simulink model "Nx8000_c"  (R2022b)
settings: Solver=VariableStepAuto  StartTime=0.0  StopTime=inf  RelTol=1e-3
libraries: instrumentseriallib x3
settings Model: Creator=twopi  LastModifiedBy=twopi

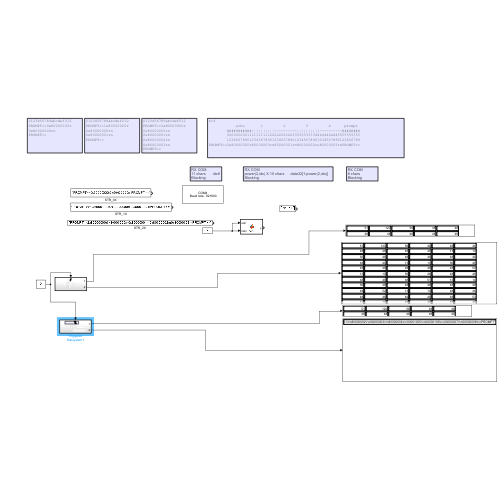
[thumbnail: Simulink's stored preview of the top-level diagram]
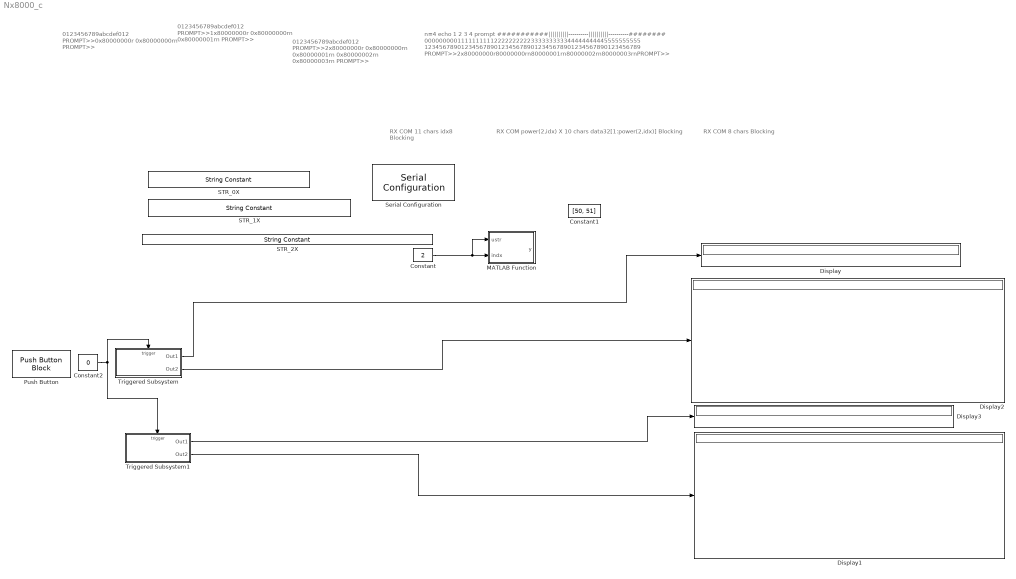
== system Nx8000_c ==
  note: RX COM
      | 11 chars       idx8
      | Blocking
  note: 0123456789abcdef012
      | PROMPT>>0x80000000r
      | 0x80000000rn
      | PROMPT>>
  note: 0123456789abcdef012
      | PROMPT>>1x80000000r
      | 0x80000000rn
      | 0x80000001rn
      | PROMPT>>
  note: 0123456789abcdef012
      | PROMPT>>2x80000000r
      | 0x80000000rn
      | 0x80000001rn
      | 0x80000002rn
      | 0x80000003rn
      | PROMPT>>
  note: n=4
      |             echo       1         2         3         4      prompt
      |         ###########||||||||||----------||||||||||----------########
      |         00000000011111111112222222222333333333344444444445555555555
      |         12345678901234567890123456789012345678901234567890123456789
      | PROMPT>>2x80000000r80000000rn80000001rn80000002rn80000003rnPROMPT>>
  note: RX COM
      | power(2,idx) X 10 chars      data32[1:power(2,idx)]
      | Blocking
  note: RX COM
      | 8 chars
      | Blocking
  Constant : Constant  Value=2  OutDataTypeStr=uint8
  Constant1 : Constant  Value=[50, 51]  OutDataTypeStr=uint8
  Constant2 : Constant  Value=0  OutDataTypeStr=uint8  SampleTime=Inf
  Display{,1..3} (4 alike) : Display
  MATLAB Function : MATLAB Function  TreatAsAtomicUnit=on
  Push Button : PushButtonBlock  OffValue=0.000000
  STR_0X : StringConstant  String="\"PROMPT>>0x80000000r0x80000000rnPROMPT>>\""
  STR_1X : StringConstant  String="\"PROMPT>>1x80000000r0x80000000rn0x80000001rnPROMPT>>\""
  STR_2X : StringConstant  String="\"PROMPT>>2x80000000r0x80000000rn0x80000001rn0x80000002rn0x80000003rnPROMPT>>\""
  Serial Configuration : instrumentseriallib/Serial Configuration  Priority=-200000  PortSel=COM4  Port=COM4  ComPort=COM4  BaudRate=921600  DataBits=8  Parity=none  StopBits=1  ByteOrder=little-endian  FlowControl=none  Timeout=10  SimulateUsing=Interpreted execution  BlockInModel=on  aMode=1
  Triggered Subsystem : Subsystem  TreatAsAtomicUnit=on
      settings: LibrarySourceBlock=|
      | hdlsllib/Ports &
      | Subsystems/Triggered
      | Subsystem
  Triggered Subsystem1 : Subsystem  TreatAsAtomicUnit=on
      settings: LibrarySourceBlock=|
      | hdlsllib/Ports &
      | Subsystems/Triggered
      | Subsystem
  wires:
  Constant/1 -> MATLAB Function/1(ustr), MATLAB Function/2(indx)
  Triggered Subsystem/1(Out1) -> Display/1
  Constant2/1 -> Triggered Subsystem1/Trigger, Triggered Subsystem/Trigger
  Triggered Subsystem1/1(Out1) -> Display3/1
  Triggered Subsystem/2(Out2) -> Display2/1
  Triggered Subsystem1/2(Out2) -> Display1/1

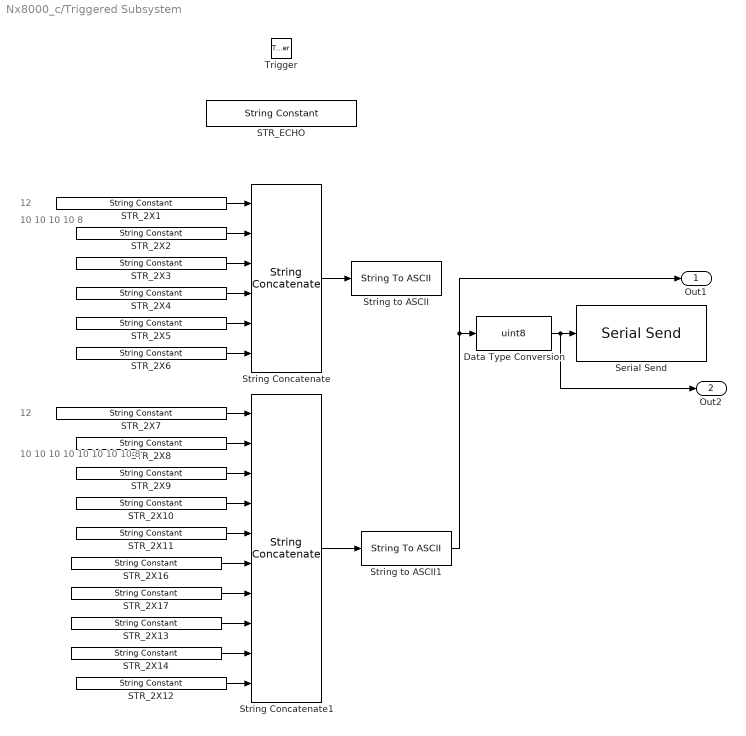
== system Nx8000_c/Triggered Subsystem ==
  note: 12
  note: 10
      |
      | 10
      |
      |
      | 10
      |
      | 10
      |
      | 8
  note: 12
  note: 10
      |
      | 10
      |
      |
      | 10
      |
      | 10
      |
      | 10
      |
      | 10
      |
      |
      | 10
      |
      | 10
      |
      | 8
  Trigger : TriggerPort  VariantControl=(inherit)
  Data Type Conversion : DataTypeConversion  OutDataTypeStr=uint8  SaturateOnIntegerOverflow=off  RndMeth=Floor
  STR_2X1 : StringConstant  String="\"2x80000000\"+char(13)+char(10)"
  STR_2X10 : StringConstant  String="\"80000003\"+char(13)+char(10)"
  STR_2X11 : StringConstant  String="\"80000004\"+char(13)+char(10)"
  STR_2X12 : StringConstant  String="\"PROMPT>>\""
  STR_2X13 : StringConstant  String="\"00000007\"+char(13)+char(10)"
  STR_2X14 : StringConstant  String="\"00000008\"+char(13)+char(10)"
  STR_2X16 : StringConstant  String="\"00001005\"+char(13)+char(10)"
  STR_2X17 : StringConstant  String="\"00000106\"+char(13)+char(10)"
  STR_2X2 : StringConstant  String="\"80000001\"+char(13)+char(10)"
  STR_2X3 : StringConstant  String="\"80000002\"+char(13)+char(10)"
  STR_2X4 : StringConstant  String="\"80000003\"+char(13)+char(10)"
  STR_2X5 : StringConstant  String="\"80000004\"+char(13)+char(10)"
  STR_2X6 : StringConstant  String="\"PROMPT>>\""
  STR_2X7 : StringConstant  String="\"3x80000000\"+char(13)+char(10)"
  STR_2X8 : StringConstant  String="\"80000001\"+char(13)+char(10)"
  STR_2X9 : StringConstant  String="\"80000002\"+char(13)+char(10)"
  STR_ECHO : StringConstant  String="\"0x8765\" + \"4321\""
  Serial Send : instrumentseriallib/Serial Send  Priority=1  PortSel=COM4  Port=COM4  ComPort=COM4  Header=[]  Terminator=Custom terminator  CustomTerminator=[62, 62]  EnableBlockingMode=on  SimulateUsing=Interpreted execution  BlockInModel=on  aMode=1
  String Concatenate : StringConcatenate  Inputs=6
  String Concatenate1 : StringConcatenate  Inputs=10
  String to ASCII : StringToASCII  OutputVectorSize=60
  String to ASCII1 : StringToASCII  OutputVectorSize=100
  Out1 : Outport
  Out2 : Outport  Port=2
  wires:
  STR_2X1/1 -> String Concatenate/1
  STR_2X2/1 -> String Concatenate/2
  STR_2X3/1 -> String Concatenate/3
  STR_2X4/1 -> String Concatenate/4
  STR_2X5/1 -> String Concatenate/5
  STR_2X6/1 -> String Concatenate/6
  Data Type Conversion/1 -> Out2/1, Serial Send/1
  STR_2X9/1 -> String Concatenate1/3
  STR_2X8/1 -> String Concatenate1/2
  STR_2X11/1 -> String Concatenate1/5
  STR_2X10/1 -> String Concatenate1/4
  STR_2X7/1 -> String Concatenate1/1
  STR_2X12/1 -> String Concatenate1/10
  STR_2X14/1 -> String Concatenate1/9
  STR_2X13/1 -> String Concatenate1/8
  STR_2X17/1 -> String Concatenate1/7
  STR_2X16/1 -> String Concatenate1/6
  String Concatenate1/1 -> String to ASCII1/1
  String to ASCII1/1 -> Out1/1, Data Type Conversion/1
  String Concatenate/1 -> String to ASCII/1

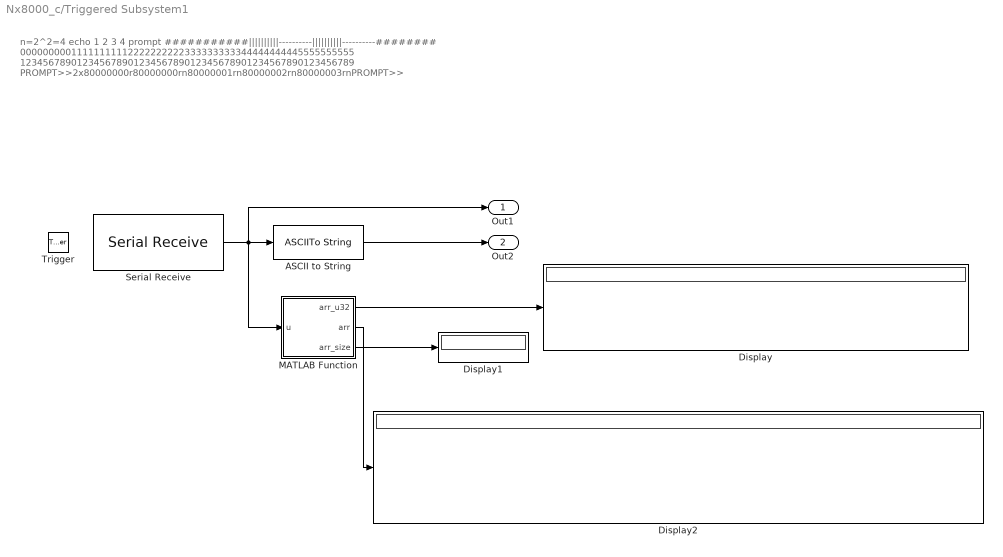
== system Nx8000_c/Triggered Subsystem1 ==
  note: n=2^2=4
      |             echo       1         2         3         4      prompt
      |         ###########||||||||||----------||||||||||----------########
      |         00000000011111111112222222222333333333344444444445555555555
      |         12345678901234567890123456789012345678901234567890123456789
      | PROMPT>>2x80000000r80000000rn80000001rn80000002rn80000003rnPROMPT>>
  Trigger : TriggerPort  TriggerType=falling  VariantControl=(inherit)
  ASCII to String : ASCIIToString
  Display : Display
  Display1 : Display
  Display2 : Display
  MATLAB Function : MATLAB Function  TreatAsAtomicUnit=on
  Serial Receive : instrumentseriallib/Serial Receive  Priority=1  PortSel=COM4  Port=COM4  ComPort=COM4  DataType=uint8  SaveDataType=uint8  ToggleHeader=off  Header=[]  ToggleTerminator=on  Terminator=Custom terminator  CustomTerminator=[62, 62]  InputFormat=Column major  ToggleDataSize=on  DataSize=[1 98]  EnableBlockingMode=on  ActionDataUnavailable=Output last received value  ActionWhenDataUnavailable=Output last received value  CustomValue=0  SampleTime=-1  SimulateUsing=Interpreted execution  BlockInModel=on  aMode=1
  Out1 : Outport
  Out2 : Outport  Port=2
  wires:
  Serial Receive/1 -> MATLAB Function/1(u), Out1/1, ASCII to String/1
  ASCII to String/1 -> Out2/1
  MATLAB Function/2(arr) -> Display2/1
  MATLAB Function/1(arr_u32) -> Display/1
  MATLAB Function/3(arr_size) -> Display1/1

== matlab function Nx8000_c/Triggered Subsystem1/MATLAB Function ==
  data: u input; arr_u32 output; arr output; arr_size output
function [arr_u32, arr, arr_size]    = fcn(u)

  nmax      = 2^8;

  arr       = zeros(nmax,8);     % create empty array of uint8 array
  arr_u32   = zeros(nmax,1);     % create empty array of uint32
  arr_size  = 2^(char(u(1))-48); % get an output arr size from ECHO (Header)

  arr_c     = char(u);           % cast input STRING into UINT8 array
  arr_u8    = uint8(arr_c);      % cast input STRING into UINT8 array

%KEEP echo  = arr_c(1,1:12);    % echo is dropped

  for i = 1 : arr_size
    arr     (i,:) = arr_u8(13+10*(i-1):20+10*(i-1)); % data only
    arr_cc        = arr_c (13+10*(i-1):20+10*(i-1)); % data only
    arr_u32 (i,1) = uint32(hex2dec(string(arr_cc))); % data only
  end

 %  arr_u32(1:arr_size,:) = arr_u32(1:nmax,:); % data only


end

== matlab function Nx8000_c/MATLAB Function ==
  data: ustr input; y output; indx input
function y = fcn(ustr, indx)

y = uint8(char(ustr));

%y = q(11:19);
